simulink model "Ausbreitungsmodell"  (R2020b)
settings: Solver=VariableStepAuto  StartTime=0.0  StopTime=100  RelTol=1e-3
model workspace (MAT data in the model file):
  k = 0.2
  s = Simulink.Parameter
  s.Value = 4
  s.DataType = 'auto'
  s.Dimensions = [1 1]
  y0 = 2e-06
settings Model: Creator=ypz  LastModifiedBy=ypz

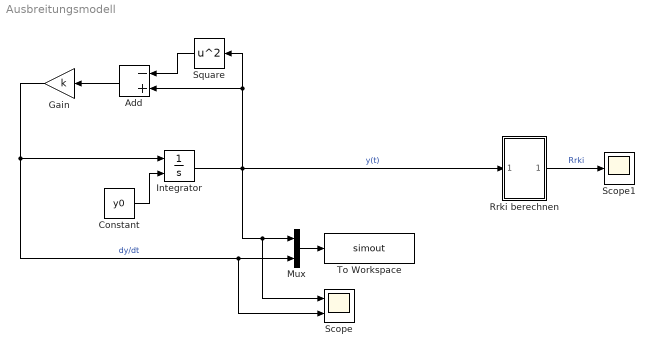
== system Ausbreitungsmodell ==
  Add : Sum  Inputs=-+
  Constant : Constant  Value=y0
  Gain : Gain  Gain=k
  Integrator : Integrator  InitialConditionSource=external
  Mux : Mux  Inputs=2
  Rrki berechnen : Subsystem
  Scope : Scope  NumInputPorts=2
  Scope1 : Scope
  Square : Math  Operator=square  SaturateOnIntegerOverflow=on
  To Workspace : ToWorkspace  VariableName=simout  SaveFormat=Timeseries  SampleTime=-1
  wires:
  Integrator/1 -> Add/2, Square/1, Rrki berechnen/1(y(t)), Scope/1, Mux/1  "y(t)"
  Constant/1 -> Integrator/2
  Square/1 -> Add/1
  Add/1 -> Gain/1
  Gain/1 -> Integrator/1, Scope/2, Mux/2  "dy/dt"
  Mux/1 -> To Workspace/1
  Rrki berechnen/1(Rrki) -> Scope1/1  "Rrki"

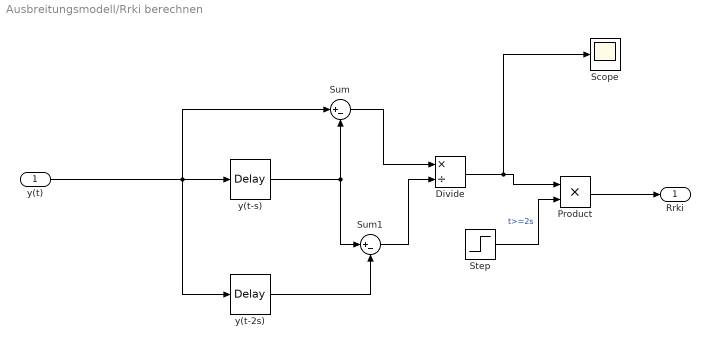
== system Ausbreitungsmodell/Rrki berechnen ==
  y(t) : Inport
  Divide : Product  Inputs=*/
  Product : Product
  Scope : Scope
  Step : Step  Time=2*s  SampleTime=0
  Sum : Sum  Inputs=|+-
  Sum1 : Sum  Inputs=|+-
  y(t-2s) : TransportDelay  DelayTime=2*s  InitialOutput=1*10*-8
  y(t-s) : TransportDelay  DelayTime=s  InitialOutput=1*10^-8
  Rrki : Outport
  wires:
  y(t-s)/1 -> Sum/2, Sum1/1
  y(t)/1 -> y(t-2s)/1, Sum/1, y(t-s)/1
  y(t-2s)/1 -> Sum1/2
  Sum/1 -> Divide/1
  Sum1/1 -> Divide/2
  Step/1 -> Product/2  "t>=2s"
  Divide/1 -> Scope/1, Product/1
  Product/1 -> Rrki/1
